simulink model "mdl01_sysIdentify"  (R2023a)
settings: Solver=FixedStepAuto  StartTime=0.0  StopTime=T1  FixedStep=Ts  RelTol=1e-3
values from neighbouring files (symbols this model uses):
  G = 3.5    [Sim01_ValidateRLS.m]
  lambda = 1    [Sim01_ValidateRLS.m]
  M = 1    [Sim01_ValidateRLS.m]
  N = 2    [Sim01_ValidateRLS.m]
  Npara = M+N+1    (= 4)    [Sim01_ValidateRLS.m]
  P0 = 1e4    (= 10000)    [Sim01_ValidateRLS.m]
  para0 = zeros(Npara,1)    [Sim01_ValidateRLS.m]
  Ts = 1e-3    (= 0.001)    [Sim01_ValidateRLS.m]
  v0 = 0    [Sim01_ValidateRLS.m]
  w0 = 2*pi*10    (= 62.8318530718)    [Sim01_ValidateRLS.m]
  wn_std = 0.1    [Sim01_ValidateRLS.m]
  x0 = 0    [Sim01_ValidateRLS.m]
  zeta = 0.3    [Sim01_ValidateRLS.m]
libraries: simulink x3
settings Model: Creator=xiaocy  LastModifiedBy=xiaocy
settings DataIOCC: SaveOutput=off  SignalLogging=off  DSMLogging=off  SaveTime=off  ReturnWorkspaceOutputs=off

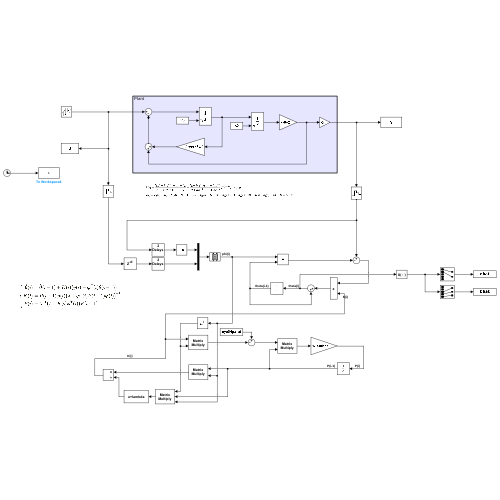
[thumbnail: Simulink's stored preview of the top-level diagram]
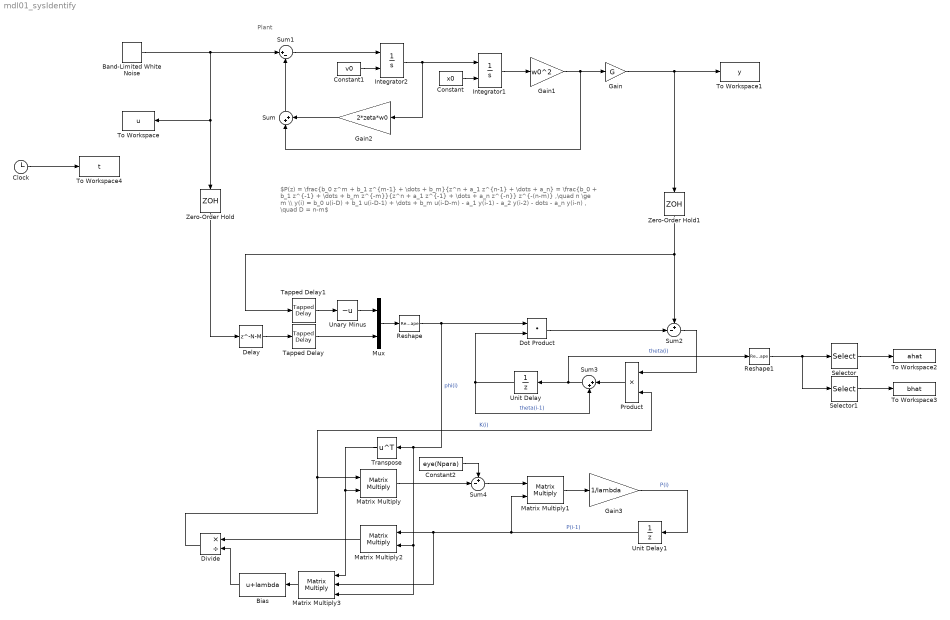
== system mdl01_sysIdentify ==
  note: $P(z) = \frac{b_0 z^m + b_1 z^{m-1} + \dots + b_m}{z^n + a_1 z^{n-1} + \dots + a_n} = \frac{b_0 + b_1 z^{-1} + \dots + b_m z^{-m}}{z^n + a_1 z^{-1} + \dots + a_n z^{-n}} z^{-(n-m)} ,\quad n \ge m \\ y(i) = b_0 u(i-D) + b_1 u(i-D-1) + \dots + b_m u(i-D-m) - a_1 y(i-1) - a_2 y(i-2) - dots - a_n y(i-n) , \quad D = n-m$
  note: Plant
  Band-Limited White Noise : simulink/Sources/Band-Limited White Noise  Cov=wn_std^2*Ts  Ts=Ts  seed=[23341]
  Bias : Bias  Bias=lambda  SaturateOnIntegerOverflow=off
  Clock : Clock
  Constant : Constant  Value=x0
  Constant1 : Constant  Value=v0
  Constant2 : Constant  Value=eye(Npara)
  Delay : Delay  DelayLength=N-M  SampleTime=Ts
  Divide : Product  Inputs=*/
  Dot Product : DotProduct  OutDataTypeStr=Inherit: Inherit via internal rule
  Gain : Gain  Gain=G
  Gain1 : Gain  Gain=w0^2
  Gain2 : Gain  Gain=2*zeta*w0
  Gain3 : Gain  Gain=1/lambda
  Integrator1 : Integrator  InitialConditionSource=external
  Integrator2 : Integrator  InitialConditionSource=external
  Matrix Multiply : Product  Multiplication=Matrix(*)
  Matrix Multiply1 : Product  Multiplication=Matrix(*)
  Matrix Multiply2 : Product  Multiplication=Matrix(*)
  Matrix Multiply3 : Product  Inputs=3  Multiplication=Matrix(*)
  Mux : Mux  Inputs=2
  Product : Product
  Reshape : Reshape  OutputDimensionality=Column vector (2-D)
  Reshape1 : Reshape
  Selector : Selector  InputPortWidth=Npara  IndexOptions=Index vector (dialog)  Indices=1:N  OutputSizes=1
  Selector1 : Selector  InputPortWidth=Npara  IndexOptions=Index vector (dialog)  Indices=N+1:Npara  OutputSizes=1
  Sum : Sum  Inputs=|++
  Sum1 : Sum  Inputs=|+-
  Sum2 : Sum  Inputs=+-|
  Sum3 : Sum  Inputs=|++
  Sum4 : Sum  Inputs=+-|
  Tapped Delay : simulink/Discrete/Tapped Delay  vinit=0.0  samptime=Ts  NumDelays=M  DelayOrder=Newest  includeCurrent=on
  Tapped Delay1 : simulink/Discrete/Tapped Delay  vinit=0.0  samptime=Ts  NumDelays=N  DelayOrder=Newest  includeCurrent=off
  To Workspace : ToWorkspace  VariableName=u  SampleTime=Ts
  To Workspace1 : ToWorkspace  VariableName=y  SampleTime=Ts
  To Workspace2 : ToWorkspace  VariableName=ahat  SampleTime=Ts
  To Workspace3 : ToWorkspace  VariableName=bhat  SampleTime=Ts
  To Workspace4 : ToWorkspace  VariableName=t  SampleTime=Ts
  Transpose : Math  Operator=transpose
  Unary Minus : UnaryMinus
  Unit Delay : UnitDelay  InitialCondition=para0  SampleTime=Ts  HasFrameUpgradeWarning=on
  Unit Delay1 : UnitDelay  InitialCondition=P0*eye(Npara)  SampleTime=Ts  HasFrameUpgradeWarning=on
  Zero-Order Hold : ZeroOrderHold  SampleTime=Ts
  Zero-Order Hold1 : ZeroOrderHold  SampleTime=Ts
  wires:
  Gain/1 -> To Workspace1/1, Zero-Order Hold1/1
  Sum/1 -> Sum1/2
  Sum1/1 -> Integrator2/1
  Gain1/1 -> Sum/1, Gain/1
  Constant/1 -> Integrator1/2
  Constant1/1 -> Integrator2/2
  Band-Limited White Noise/1 -> Sum1/1, Zero-Order Hold/1, To Workspace/1
  Integrator2/1 -> Gain2/1, Integrator1/1
  Gain2/1 -> Sum/2
  Integrator1/1 -> Gain1/1
  Delay/1 -> Tapped Delay/1
  Zero-Order Hold/1 -> Delay/1
  Zero-Order Hold1/1 -> Tapped Delay1/1, Sum2/1
  Mux/1 -> Reshape/1
  Tapped Delay1/1 -> Unary Minus/1
  Tapped Delay/1 -> Mux/2
  Unary Minus/1 -> Mux/1
  Unit Delay/1 -> Sum3/2, Dot Product/2  "theta(i-1)"
  Sum3/1 -> Reshape1/1, Unit Delay/1  "theta(i)"
  Dot Product/1 -> Sum2/2
  Product/1 -> Sum3/1
  Sum2/1 -> Product/1
  Divide/1 -> Matrix Multiply/1, Product/2  "K(i)"
  Gain3/1 -> Unit Delay1/1  "P(i)"
  Unit Delay1/1 -> Matrix Multiply3/2, Matrix Multiply2/1, Matrix Multiply1/2  "P(i-1)"
  Reshape/1 -> Matrix Multiply3/3, Matrix Multiply2/2, Transpose/1, Dot Product/1  "phi(i)"
  Transpose/1 -> Matrix Multiply3/1, Matrix Multiply/2
  Matrix Multiply/1 -> Sum4/2
  Constant2/1 -> Sum4/1
  Sum4/1 -> Matrix Multiply1/1
  Matrix Multiply1/1 -> Gain3/1
  Matrix Multiply3/1 -> Bias/1
  Matrix Multiply2/1 -> Divide/1
  Bias/1 -> Divide/2
  Selector/1 -> To Workspace2/1
  Selector1/1 -> To Workspace3/1
  Reshape1/1 -> Selector1/1, Selector/1
  Clock/1 -> To Workspace4/1
